simulink model "TwoDronesCollision"  (R2018b)
settings: Solver=VariableStepAuto  StartTime=0.0  StopTime=10.0  RelTol=1e-3
undefined symbols (not defined in the file or in its folder): bx, by, ConflictDrone2andDrone4, deltaVx2, deltaVx4, deltaVy2, deltaVy4, m, VelocityStarX2, VelocityStarX4, VelocityStarY2, VelocityStarY4, vx20, vx40, vy20, vy40, x20, x40, y20, y40
libraries: simulink x4
settings Model: Creator=CowUser  LastModifiedBy=CowUser

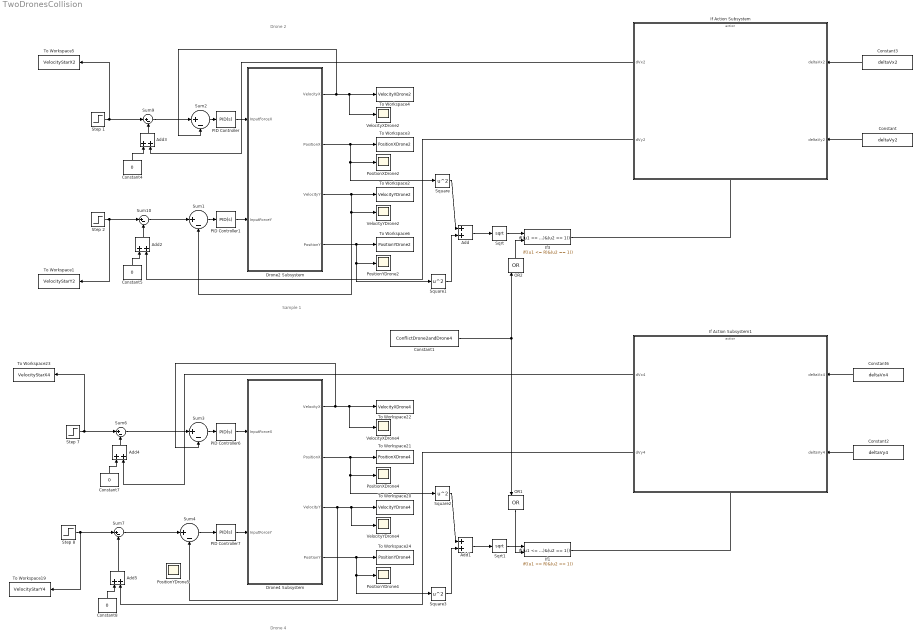
== system TwoDronesCollision ==
  note: Drone 4
  note: Sample 1
  note: Drone 2
  Add{,1..5} (6 alike) : Sum
  Constant : Constant  Value=deltaVy2
  Constant1 : Constant  Value=ConflictDrone2andDrone4
  Constant2 : Constant  Value=deltaVy4
  Constant3 : Constant  Value=deltaVx2
  Constant{4..5,7..8} (4 alike) : Constant  Value=0
  Constant6 : Constant  Value=deltaVx4
  "Drone2 Subsystem " : Subsystem
  "Drone4 Subsystem " : Subsystem
  If Action Subsystem : Subsystem  TreatAsAtomicUnit=on
  If Action Subsystem1 : Subsystem  TreatAsAtomicUnit=on
  If1 : If  NumInputs=2  IfExpression=(u1 <= R)&(u2 == 1)  ShowElse=off
  If3 : If  NumInputs=2  IfExpression=(u1 <= R)&(u2 == 1)  ShowElse=off
  OR1 : Logic  Operator=OR  Inputs=3  IconShape=distinctive  AllPortsSameDT=off  OutDataTypeStr='double'
  OR2 : Logic  Operator=OR  Inputs=3  IconShape=distinctive  AllPortsSameDT=off  OutDataTypeStr='double'
  PID Controller{,1,6..7} (4 alike) : simulink/Continuous/PID Controller  Controller=PID  Form=Parallel  TimeDomain=Continuous-time  SampleTime=-1  IntegratorMethod=Forward Euler  FilterMethod=Forward Euler  ControllerParametersSource=internal  P=800  I=40  D=1  UseFilter=on  N=100  TunerSelectOption=Transfer Function Based (PID Tuner App)  InitialConditionSource=internal  InitialConditionForIntegrator=0  InitialConditionForFilter=0  DifferentiatorICPrevScaledInput=0  ExternalReset=none  TrackingMode=off  Kt=1  LimitOutput=off  UpperSaturationLimit=inf  LowerSaturationLimit=-inf  LinearizeAsGain=on  AntiWindupMode=none  Kb=1  POutMin=[]  POutMax=[]  IOutMin=[]  IOutMax=[]  DOutMin=[]  DOutMax=[]  NOutMin=[]  NOutMax=[]  SumOutMin=[]  SumOutMax=[]  SaturationOutMin=[]  SaturationOutMax=[]  PParamMin=[]  PParamMax=[]  IParamMin=[]  IParamMax=[]  DParamMin=[]  DParamMax=[]  NParamMin=[]  NParamMax=[]  KbParamMin=[]  KbParamMax=[]  KtParamMin=[]  KtParamMax=[]  KbOutMin=[]  KbOutMax=[]  KtOutMin=[]  KtOutMax=[]  IntegratorOutMin=[]  IntegratorOutMax=[]  FilterOutMin=[]  FilterOutMax=[]  SumI1OutMin=[]  SumI1OutMax=[]  SumI2OutMin=[]  SumI2OutMax=[]  SumI3OutMin=[]  SumI3OutMax=[]  SumI4OutMin=[]  SumI4OutMax=[]  SumDOutMin=[]  SumDOutMax=[]  DifferentiatorOutMin=[]  DifferentiatorOutMax=[]  FilterDiffOutCoefMin=[]  FilterDiffOutCoefMax=[]  ReciprocalOutMin=[]  ReciprocalOutMax=[]  SumDenOutMin=[]  SumDenOutMax=[]  SumNumOutMin=[]  SumNumOutMax=[]  DivideOutMin=[]  DivideOutMax=[]  IntegratorContinuousStateAttributes=''  IntegratorStateMustResolveToSignalObject=off  IntegratorRTWStateStorageClass=Auto  FilterContinuousStateAttributes=''  FilterStateMustResolveToSignalObject=off  FilterRTWStateStorageClass=Auto  ParallelPVariant=InternalParameters  IdealPVariant=Disabled  IVariant=InternalParameters  DVariant=InternalParameters  IntegratorVariant=Continuous  SatVariant=Disabled  AWVariant=Passthrough  PCopyVariant=Disabled  TRVariant=Disabled  FdbkBlocksVariant=Forward  IdealPFdbkVariant=Disabled  SatFdbkVariant=Disabled  DerivativeFilterVariant=ContFilter  NVariant=InternalParameters  NCopyVariant=Disabled  FilterICVariant=InternalICsFilter  IntegratorICVariant=InternalICs  ExternalResetVariant=Disabled  TRSumVariant=Passthrough  SumFdbkVariant=Disabled  SumVariant=Sum_PID
  PositionXDrone2 : Scope
  PositionXDrone4 : Scope
  PositionYDrone2 : Scope
  PositionYDrone4 : Scope
  PositionYDrone5 : Scope
  Sqrt : Sqrt  SaturateOnIntegerOverflow=on
  Sqrt1 : Sqrt  SaturateOnIntegerOverflow=on
  Square{,1..3} (4 alike) : Math  Operator=square  SaturateOnIntegerOverflow=on
  Step 1 : Step  Time=0  After=VelocityStarX2  SampleTime=0
  Step 2 : Step  Time=0  After=VelocityStarY2  SampleTime=0
  Step 7 : Step  Time=0  After=VelocityStarX4  SampleTime=0
  Step 8 : Step  Time=0  After=VelocityStarY4  SampleTime=0
  Sum{1..4,6..7,9..10} (8 alike) : Sum  Inputs=|+-
  To Workspace1 : ToWorkspace  VariableName=VelocityStarY2  SampleTime=-1
  To Workspace19 : ToWorkspace  VariableName=VelocityStarY4  SampleTime=-1
  To Workspace2 : ToWorkspace  VariableName=VelocityYDrone2  SampleTime=-1
  To Workspace20 : ToWorkspace  VariableName=VelocityYDrone4  SampleTime=-1
  To Workspace21 : ToWorkspace  VariableName=PositionXDrone4  SampleTime=-1
  To Workspace22 : ToWorkspace  VariableName=VelocityXDrone4  SampleTime=-1
  To Workspace23 : ToWorkspace  VariableName=VelocityStarX4  SampleTime=-1
  To Workspace24 : ToWorkspace  VariableName=PositionYDrone4  SampleTime=-1
  To Workspace3 : ToWorkspace  VariableName=PositionXDrone2  SampleTime=-1
  To Workspace4 : ToWorkspace  VariableName=VelocityXDrone2  SampleTime=-1
  To Workspace5 : ToWorkspace  VariableName=VelocityStarX2  SampleTime=-1
  To Workspace6 : ToWorkspace  VariableName=PositionYDrone2  SampleTime=-1
  VelocityXDrone2 : Scope
  VelocityXDrone4 : Scope
  VelocityYDrone2 : Scope
  VelocityYDrone4 : Scope
  wires:
  OR1/1 -> If1/2
  Sum9/1 -> Sum2/1
  Sum3/1 -> PID Controller6/1
  If Action Subsystem/1(dVx2) -> Add3/2
  If3/1 -> If Action Subsystem/Action
  OR2/1 -> If3/2
  Constant5/1 -> Add2/1
  Step 8/1 -> To Workspace19/1, Sum7/1
  Constant1/1 -> OR1/1, OR2/1
  PID Controller/1 -> "Drone2 Subsystem "/1(InputForceX)
  Step 2/1 -> Sum10/1, To Workspace1/1
  "Drone4 Subsystem "/4(PositionY) -> Square3/1, PositionYDrone4/1, To Workspace24/1
  Sum2/1 -> PID Controller/1
  "Drone2 Subsystem "/4(PositionY) -> Square1/1, PositionYDrone2/1, To Workspace6/1
  "Drone4 Subsystem "/1(VelocityX) -> Sum3/2, To Workspace22/1, VelocityXDrone4/1
  PID Controller1/1 -> "Drone2 Subsystem "/2(InputForceY)
  Add/1 -> Sqrt/1
  Add3/1 -> Sum9/2
  Constant4/1 -> Add3/1
  Constant7/1 -> Add4/1
  Add2/1 -> Sum10/2
  Add4/1 -> Sum6/2
  Sum4/1 -> PID Controller7/1
  "Drone4 Subsystem "/2(PositionX) -> Square2/1, PositionXDrone4/1, To Workspace21/1
  Square3/1 -> Add1/2
  "Drone2 Subsystem "/2(PositionX) -> Square/1, PositionXDrone2/1, To Workspace3/1
  Sum10/1 -> Sum1/1
  Sqrt1/1 -> If1/1
  Constant8/1 -> Add5/1
  Square/1 -> Add/1
  Add1/1 -> Sqrt1/1
  Sum1/1 -> PID Controller1/1
  Sqrt/1 -> If3/1
  Square1/1 -> Add/2
  If Action Subsystem1/2(dVy4) -> Add5/2
  Step 1/1 -> Sum9/1, To Workspace5/1
  Square2/1 -> Add1/1
  If Action Subsystem1/1(dVx4) -> Add4/2
  "Drone4 Subsystem "/3(VelocityY) -> Sum4/2, VelocityYDrone4/1, To Workspace20/1
  "Drone2 Subsystem "/1(VelocityX) -> VelocityXDrone2/1, To Workspace4/1, Sum2/2
  Step 7/1 -> Sum6/1, To Workspace23/1
  "Drone2 Subsystem "/3(VelocityY) -> Sum1/2, VelocityYDrone2/1, To Workspace2/1
  Sum7/1 -> Sum4/1
  If Action Subsystem/2(dVy2) -> Add2/2
  PID Controller6/1 -> "Drone4 Subsystem "/1(InputForceX)
  If1/1 -> If Action Subsystem1/Action
  Add5/1 -> Sum7/2
  PID Controller7/1 -> "Drone4 Subsystem "/2(InputForceY)
  Sum6/1 -> Sum3/1
  Constant2/1 -> If Action Subsystem1/2(deltaVy4)
  Constant6/1 -> If Action Subsystem1/1(deltaVx4)
  Constant3/1 -> If Action Subsystem/1(deltaVx2)
  Constant/1 -> If Action Subsystem/2(deltaVy2)

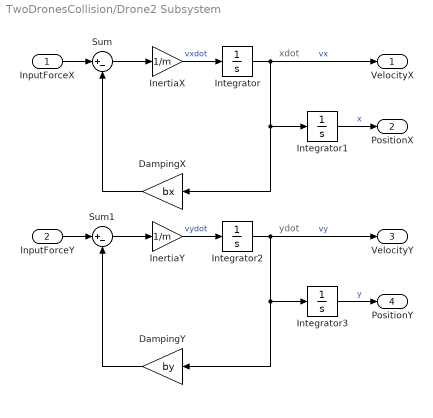
== system TwoDronesCollision/Drone2 Subsystem  ==
  note: xdot
  note: ydot
  InputForceX : Inport
  InputForceY : Inport  Port=2
  "DampingX " : Gain  Gain=bx
  DampingY : Gain  Gain=by
  InertiaX : Gain  Gain=1/m
  InertiaY : Gain  Gain=1/m
  Integrator : Integrator  InitialCondition=vx20
  Integrator1 : Integrator  InitialCondition=x20
  Integrator2 : Integrator  InitialCondition=vy20
  Integrator3 : Integrator  InitialCondition=y20
  Sum : Sum  Inputs=|+-
  Sum1 : Sum  Inputs=|+-
  VelocityX : Outport
  PositionX : Outport  Port=2
  VelocityY : Outport  Port=3
  PositionY : Outport  Port=4
  wires:
  InputForceX/1 -> Sum/1
  InertiaX/1 -> Integrator/1  "vxdot"
  Sum/1 -> InertiaX/1
  Integrator/1 -> VelocityX/1, Integrator1/1, "DampingX "/1  "vx"
  "DampingX "/1 -> Sum/2
  Integrator1/1 -> PositionX/1  "x"
  DampingY/1 -> Sum1/2
  Sum1/1 -> InertiaY/1
  InertiaY/1 -> Integrator2/1  "vydot"
  Integrator3/1 -> PositionY/1  "y"
  InputForceY/1 -> Sum1/1
  Integrator2/1 -> VelocityY/1, Integrator3/1, DampingY/1  "vy"

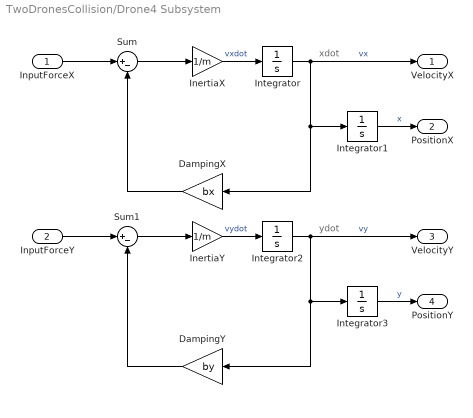
== system TwoDronesCollision/Drone4 Subsystem  ==
  note: xdot
  note: ydot
  InputForceX : Inport
  InputForceY : Inport  Port=2
  "DampingX " : Gain  Gain=bx
  DampingY : Gain  Gain=by
  InertiaX : Gain  Gain=1/m
  InertiaY : Gain  Gain=1/m
  Integrator : Integrator  InitialCondition=vx40
  Integrator1 : Integrator  InitialCondition=x40
  Integrator2 : Integrator  InitialCondition=vy40
  Integrator3 : Integrator  InitialCondition=y40
  Sum : Sum  Inputs=|+-
  Sum1 : Sum  Inputs=|+-
  VelocityX : Outport
  PositionX : Outport  Port=2
  VelocityY : Outport  Port=3
  PositionY : Outport  Port=4
  wires:
  InertiaX/1 -> Integrator/1  "vxdot"
  Integrator/1 -> VelocityX/1, Integrator1/1, "DampingX "/1  "vx"
  "DampingX "/1 -> Sum/2
  Integrator1/1 -> PositionX/1  "x"
  DampingY/1 -> Sum1/2
  InertiaY/1 -> Integrator2/1  "vydot"
  Integrator3/1 -> PositionY/1  "y"
  Integrator2/1 -> VelocityY/1, Integrator3/1, DampingY/1  "vy"
  InputForceX/1 -> Sum/1
  InputForceY/1 -> Sum1/1
  Sum1/1 -> InertiaY/1
  Sum/1 -> InertiaX/1

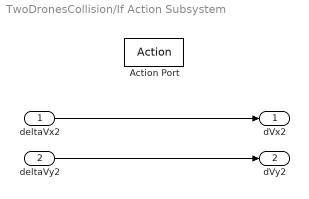
== system TwoDronesCollision/If Action Subsystem ==
  deltaVx2 : Inport
  deltaVy2 : Inport  Port=2
  Action Port : ActionPort  ActionType=then
  dVx2 : Outport
  dVy2 : Outport  Port=2
  wires:
  deltaVx2/1 -> dVx2/1
  deltaVy2/1 -> dVy2/1

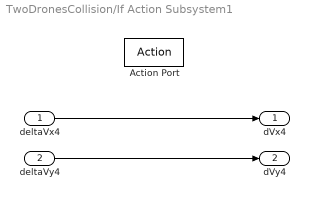
== system TwoDronesCollision/If Action Subsystem1 ==
  deltaVx4 : Inport
  deltaVy4 : Inport  Port=2
  Action Port : ActionPort  ActionType=then
  dVx4 : Outport
  dVy4 : Outport  Port=2
  wires:
  deltaVx4/1 -> dVx4/1
  deltaVy4/1 -> dVy4/1
